simulink model "motorsim"  (R2015b)
settings: Solver=ode4  StartTime=0.0  StopTime=10  FixedStep=0.001  RelTol=1e-3
undefined symbols (not defined in the file or in its folder): Beq, Jeq, Ka, Kb, Kg, qc_get_step_size, Rm
libraries: quarc_library x4
settings Model: SimulationMode=external  ExtModeTrigDuration=10000  Creator=millerid  LastModifiedBy=flynng
settings SolverCC: PositivePriorityOrder=on
settings RTWCC: SystemTargetFile=quarc_win64.tlc  TemplateMakefile=quarc_default_tmf  Description=QUARC Win64 Target
settings STFCustomTargetCC: TargetPreCompLibLocation=C:\ProgramData\QUARC\lib\2015b\win64\release  GeneratePreprocessorConditionals=Use local settings  MatFileLogging=on  CPPClassGenCompliant=off
settings GRTTargetCC: TargetPreCompLibLocation=C:\ProgramData\QUARC\lib\2015b\win64\release  ParMdlRefBuildCompliant=off  CompOptLevelCompliant=off  CombineOutputUpdateFcns=off  CPPClassGenCompliant=off  GRTInterface=on  UseToolchainInfoCompliant=off  ExtMode=on  ExtModeMexFile=quarc_comm

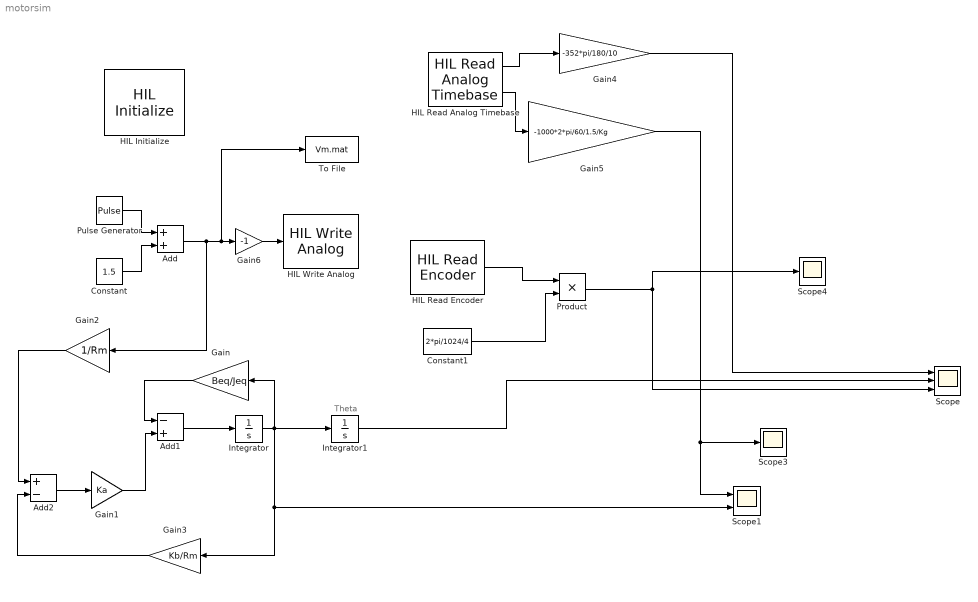
== system motorsim ==
  note: Theta
  Add : Sum
  Add1 : Sum  Inputs=-+
  Add2 : Sum  Inputs=+-
  Constant : Constant  Value=1.5
  Constant1 : Constant  Value=2*pi/1024/4
  Gain : Gain  Gain=Beq/Jeq
  Gain1 : Gain  Gain=Ka
  Gain2 : Gain  Gain=1/Rm
  Gain3 : Gain  Gain=Kb/Rm
  Gain4 : Gain  Gain=-352*pi/180/10
  Gain5 : Gain  Gain=-1000*2*pi/60/1.5/Kg
  Gain6 : Gain  Gain=-1
  HIL Initialize : quarc_library/Data Acquisition/Generic/Configuration/HIL Initialize  Priority=-99  object_name=controller  board_type=q8_usb  board_number=0  board_options=update_rate=normal;decimation=1  exclusive=off  active=off  hardware_clocks=[0:2]  clock_modes=[]  initial_clock_frequencies=[]  set_clock_params_at_start=off  set_clock_params_at_switch_in=off  set_clock_frequencies_at_start=off  set_clock_frequencies_at_switch_in=off  analog_input_channels=[0:7]  analog_input_maximums=10  analog_input_minimums=-10  set_analog_input_params_at_start=on  set_analog_input_params_at_switch_in=off  analog_output_channels=[0:7]  analog_output_maximums=10  analog_output_minimums=-10  initial_analog_outputs=[0]  final_analog_outputs=[0]  watchdog_analog_outputs=0  set_analog_output_params_at_start=on  set_analog_output_params_at_switch_in=off  set_analog_outputs_at_start=on  set_analog_outputs_at_switch_in=off  set_analog_outputs_at_terminate=on  set_analog_outputs_at_switch_out=off  set_analog_outputs_on_watchdog=off  digital_input_channels=[]  digital_output_channels=[]  digital_output_configuration=[]  initial_digital_outputs=[1]  final_digital_outputs=[1]  watchdog_digital_outputs=[1]  set_digital_output_params_at_start=off  set_digital_output_params_at_switch_in=off  set_digital_outputs_at_start=on  set_digital_outputs_at_switch_in=off  set_digital_outputs_at_terminate=on  set_digital_outputs_at_switch_out=off  set_digital_outputs_on_watchdog=off  encoder_channels=[0:7]  quadrature=[4]  encoder_filter_frequency=[]  initial_encoder_counts=[0]  set_encoder_params_at_start=on  set_encoder_params_at_switch_in=off  set_encoder_counts_at_start=on  set_encoder_counts_at_switch_in=off  pwm_channels=[0:7]  pwm_modes=0  pwm_frequency=99.532799999999995e6/4095  pwm_configuration=[0]  pwm_alignment=[0]  pwm_polarity=[1]  pwm_leading_deadband=[0]  pwm_trailing_deadband=[0]  initial_pwm_outputs=[0]  final_pwm_outputs=[0]  watchdog_pwm_outputs=[0]  set_pwm_params_at_start=on  set_pwm_params_at_switch_in=off  set_pwm_outputs_at_start=on  set_pwm_outputs_at_switch_in=off  set_pwm_outputs_at_terminate=on  set_pwm_outputs_at_switch_out=off  set_pwm_outputs_on_watchdog=off  other_output_channels=[]  initial_other_outputs=[]  final_other_outputs=[]  watchdog_other_outputs=[]  set_other_outputs_at_start=off  set_other_outputs_at_switch_in=off  set_other_outputs_at_terminate=off  set_other_outputs_at_switch_out=off  set_other_outputs_on_watchdog=off
  HIL Read Analog Timebase : quarc_library/Data Acquisition/Generic/Timebases/HIL Read Analog Timebase  object_name=controller  clock=0  channels=[0:1]  samples_in_buffer=max(ceil(1/qc_get_step_size), 1)  active=on  vector_output=off
      settings: AttributesFormatString=(%<object_name>)
  HIL Read Encoder : quarc_library/Data Acquisition/Generic/Immediate I//O/HIL Read Encoder  object_name=controller  channels=0  sample_time=qc_get_step_size  active=on  vector_output=off  data_type_mode=Inherit via back propagation  data_type=double
  HIL Write Analog : quarc_library/Data Acquisition/Generic/Immediate I//O/HIL Write Analog  object_name=controller  channels=0  sample_time=-1  active=off  vector_input=off
  Integrator : Integrator
  Integrator1 : Integrator
  Product : Product
  Pulse Generator : DiscretePulseGenerator  PulseType=Time based  Amplitude=2  Period=2.5  PulseWidth=50
  Scope : Scope  NumInputPorts=3
  Scope1 : Scope  NumInputPorts=2
  Scope3 : Scope
  Scope4 : Scope
  To File : ToFile  Filename=Vm.mat  MatrixName=Vm
  wires:
  Constant/1 -> Add/2
  Pulse Generator/1 -> Add/1
  Add/1 -> To File/1, Gain6/1, Gain2/1
  Constant1/1 -> Product/2
  HIL Read Encoder/1 -> Product/1
  HIL Read Analog Timebase/1 -> Gain4/1
  HIL Read Analog Timebase/2 -> Gain5/1
  Add1/1 -> Integrator/1
  Integrator/1 -> Integrator1/1, Gain/1, Gain3/1, Scope1/2
  Gain/1 -> Add1/1
  Gain1/1 -> Add1/2
  Add2/1 -> Gain1/1
  Gain2/1 -> Add2/1
  Gain3/1 -> Add2/2
  Integrator1/1 -> Scope/2
  Gain4/1 -> Scope/1
  Gain5/1 -> Scope1/1, Scope3/1
  Product/1 -> Scope4/1, Scope/3
  Gain6/1 -> HIL Write Analog/1
